simulink model "esempio0S"  (R2021a)
settings: Solver=VariableStepAuto  StartTime=0.0  StopTime=10.0  RelTol=1e-3
values from neighbouring files (symbols this model uses):
  A = -5    [esempio0.m]    (also in esercizio.m = [-1 -2; 1 -1]; esercizio2.m = [0 2; -10 -12]; esercizio3.m = [0 1; -5 -1]; esercizio4.m = [-7 1; -12 0])
  B = 1    [esempio0.m]    (also in esercizio.m = [0;1]; esercizio2.m = [0;1]; esercizio3.m = [0;1]; esercizio4.m = [0;1])
  C = 1    [esempio0.m]    (also in esercizio.m = [1 0;0 1]; esercizio2.m = [1 0;0 1]; esercizio3.m = [1 0; 0 1]; esercizio4.m = [1 0; 0 1])
  D = 0    [esempio0.m]    (also in esercizio.m = zeros(2,1); esercizio2.m = zeros(2,1); esercizio3.m = zeros(2,1); esercizio4.m = zeros(2,1))
  K = place(A, B, P)    [esempio0.m]    (also in esercizio.m; esercizio2.m; esercizio3.m; esercizio4.m)
  x0 = 0    [esempio0.m]    (also in esercizio2.m = [0;0]; esercizio3.m = [0;0]; esercizio4.m = [0;0])
settings Model: Creator=itama  LastModifiedBy=itama
settings SolverCC: AlgebraicLoopSolver=TrustRegion
settings DebuggingCC: SFMachineParentedDataDiag=warning

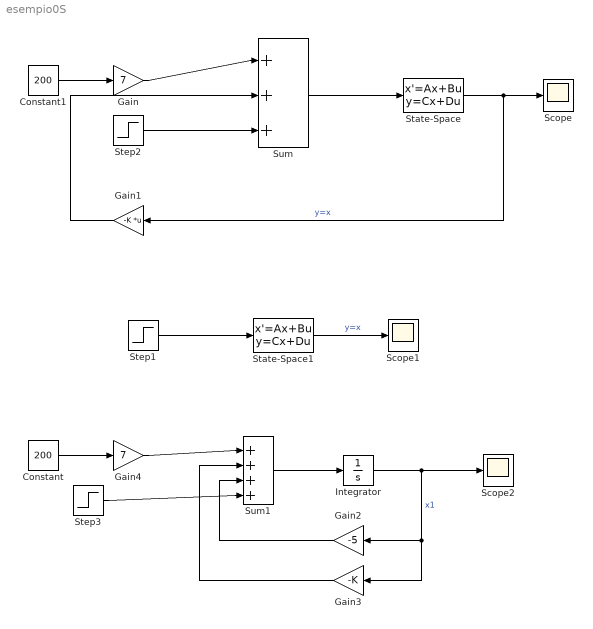
== system esempio0S ==
  Constant : Constant  Value=200
  Constant1 : Constant  Value=200
  Gain : Gain  Gain=7
  Gain1 : Gain  Gain=-K  Multiplication=Matrix(K*u)
  Gain2 : Gain  Gain=-5
  Gain3 : Gain  Gain=-K
  Gain4 : Gain  Gain=7
  Integrator : Integrator
  Scope : Scope
  Scope1 : Scope
  Scope2 : Scope
  State-Space : StateSpace  A=A  B=B  C=C  D=D  InitialCondition=x0
  State-Space1 : StateSpace  A=A  B=B  C=C  D=D  InitialCondition=x0
  Step1 : Step  Time=0  SampleTime=0
  Step2 : Step  Time=0  SampleTime=0
  Step3 : Step  Time=0  SampleTime=0
  Sum : Sum  Inputs=|+++
  Sum1 : Sum  Inputs=|++++
  wires:
  Gain/1 -> Sum/1
  Sum/1 -> State-Space/1
  State-Space/1 -> Gain1/1, Scope/1  "y=x"
  Gain1/1 -> Sum/2
  Step1/1 -> State-Space1/1
  State-Space1/1 -> Scope1/1  "y=x"
  Integrator/1 -> Gain3/1, Gain2/1, Scope2/1  "x1"
  Sum1/1 -> Integrator/1
  Gain2/1 -> Sum1/3
  Gain3/1 -> Sum1/2
  Gain4/1 -> Sum1/1
  Constant/1 -> Gain4/1
  Step2/1 -> Sum/3
  Step3/1 -> Sum1/4
  Constant1/1 -> Gain/1
